simulink model "simulator"  (R2020b)
settings: Solver=FixedStepAuto  StartTime=0.0  StopTime=t_end  FixedStep=0.01  RelTol=1e-3
values from neighbouring files (symbols this model uses):
  A = zeros(6,6)    [main_simulator.m]    (also in main_simulatorTOF.m)
  B = zeros(6,3)    [main_simulator.m]    (also in main_simulatorTOF.m)
  C = zeros(3,6)    [main_simulator.m]    (also in main_simulatorTOF.m)
  D = zeros(3,3)    [main_simulator.m]    (also in main_simulatorTOF.m)
  d_input = 0*1    (= 0)    [main_simulator.m]    (also in main_simulatorTOF.m = 1)
  d_sensor = 0    [main_simulator.m]    (also in main_simulatorTOF.m)
  I = m*Rbot*Rbot/2    (= 0.3125)    [main_simulator.m]    (also in main_simulatorTOF.m)
  Kdth = 5    [main_simulator.m]    (also in main_simulatorTOF.m)
  Kdx = 80    [main_simulator.m]    (also in main_simulatorTOF.m)
  Kdy = 60    [main_simulator.m]    (also in main_simulatorTOF.m)
  Kpth = 20    [main_simulator.m]    (also in main_simulatorTOF.m)
  Kpx = 25    [main_simulator.m]    (also in main_simulatorTOF.m)
  Kpy = 10    [main_simulator.m]    (also in main_simulatorTOF.m)
  m = 10    [main_simulator.m]    (also in main_simulatorTOF.m)
  Rdist = Lw + xset    (= 0.5)    [main_simulator.m]    (also in main_simulatorTOF.m)
  X0 = zeros(6,1)    [main_simulator.m]    (also in main_simulatorTOF.m)
undefined symbols (not defined in the file or in its folder): magnitude, sigbuilder_block
libraries: simulink x3
settings Model: Creator=danny  LastModifiedBy=danny
settings SolverCC: AlgebraicLoopSolver=Auto
settings DebuggingCC: SFMachineParentedDataDiag=error

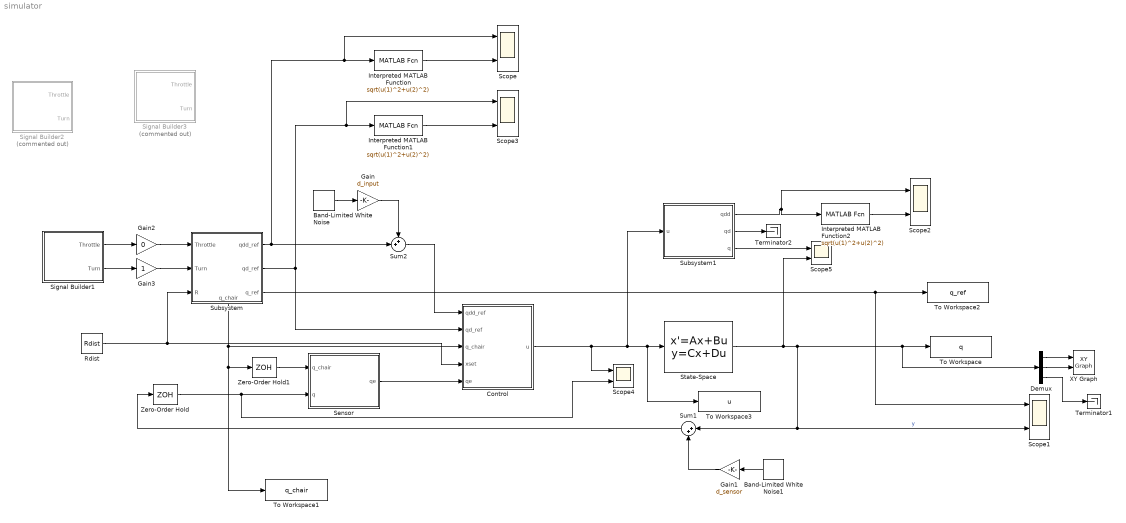
== system simulator ==
  Band-Limited White Noise : simulink/Sources/Band-Limited White Noise  Cov=[0.001]  Ts=0.1  seed=[23341]
  Band-Limited White Noise1 : simulink/Sources/Band-Limited White Noise  Cov=[0.0001]  Ts=0.15  seed=[23341]
  Control : Subsystem
  Demux : Demux  Outputs=3
  Gain : Gain  Gain=d_input
  Gain1 : Gain  Gain=d_sensor
  Gain2 : Gain  Gain=0
  Gain3 : Gain
  Interpreted MATLAB Function : MATLABFcn  MATLABFcn=sqrt(u(1)^2+u(2)^2)
  Interpreted MATLAB Function1 : MATLABFcn  MATLABFcn=sqrt(u(1)^2+u(2)^2)
  Interpreted MATLAB Function2 : MATLABFcn  MATLABFcn=sqrt(u(1)^2+u(2)^2)
  Rdist : Constant  Value=Rdist
  Scope{,1..5} (6 alike) : Scope  NumInputPorts=2
  Sensor : Subsystem
  Signal Builder1 : Subsystem  Tag=STV Subsys  LoadFcn=sigbuilder_block('load');  StartFcn=sigbuilder_block('start');  StopFcn=sigbuilder_block('stop');  ClipboardFcn=sigbuilder_block('clipboard');  mask(Sigbuilder block){tuvar=[0:10]}
      mask help: Simulink:masks:SigbuilderBlock_MD
      mask init:
      | if ~strcmp(get_param(bdroot(gcbh),'SimulationStatus'),'stopped') tuvar = sigbuilder_block('maskInit'); end
      settings: CopyFcn=sigbuilder_block('copy');  DeleteFcn=sigbuilder_block('delete');  ModelCloseFcn=sigbuilder_block('modelClose');  PreSaveFcn=sigbuilder_block('preSave');  PauseFcn=sigbuilder_block('pause');  ContinueFcn=sigbuilder_block('continue');  NameChangeFcn=sigbuilder_block('namechange');  OpenFcn=sigbuilder_block('open',[1440 169 815 516 ]);  CloseFcn=sigbuilder_block('close');
      mask Display: plot(0, 0, 100, 100,[2, 2, 32, 32, 2], [68, 8, 8, 68, 68],[32, 2], [38, 38], [32, 19, 2],[53, 60, 44], [32, 17, 17, 2],[16, 16, 31, 31]);txt = getActiveGroup(gcbh);text(2, 100, txt,'verticalAlignment', 'top');
  Signal Builder2 : Subsystem  Tag=STV Subsys  Commented=on  LoadFcn=sigbuilder_block('load');  StartFcn=sigbuilder_block('start');  StopFcn=sigbuilder_block('stop');  ClipboardFcn=sigbuilder_block('clipboard');  mask(Sigbuilder block){tuvar=[0:10]}
      mask help: Simulink:masks:SigbuilderBlock_MD
      mask init:
      | if ~strcmp(get_param(bdroot(gcbh),'SimulationStatus'),'stopped') tuvar = sigbuilder_block('maskInit'); end
      settings: CopyFcn=sigbuilder_block('copy');  DeleteFcn=sigbuilder_block('delete');  ModelCloseFcn=sigbuilder_block('modelClose');  PreSaveFcn=sigbuilder_block('preSave');  PauseFcn=sigbuilder_block('pause');  ContinueFcn=sigbuilder_block('continue');  NameChangeFcn=sigbuilder_block('namechange');  OpenFcn=sigbuilder_block('open',[87 196 1164 589 ]);  CloseFcn=sigbuilder_block('close');
      mask Display: plot(0, 0, 100, 100,[2, 2, 32, 32, 2], [68, 8, 8, 68, 68],[32, 2], [38, 38], [32, 19, 2],[53, 60, 44], [32, 17, 17, 2],[16, 16, 31, 31]);txt = getActiveGroup(gcbh);text(2, 100, txt,'verticalAlignment', 'top');
  Signal Builder3 : Subsystem  Tag=STV Subsys  Commented=on  LoadFcn=sigbuilder_block('load');  StartFcn=sigbuilder_block('start');  StopFcn=sigbuilder_block('stop');  ClipboardFcn=sigbuilder_block('clipboard');  mask(Sigbuilder block){tuvar=[0:10]}
      mask help: Simulink:masks:SigbuilderBlock_MD
      mask init:
      | if ~strcmp(get_param(bdroot(gcbh),'SimulationStatus'),'stopped') tuvar = sigbuilder_block('maskInit'); end
      settings: CopyFcn=sigbuilder_block('copy');  DeleteFcn=sigbuilder_block('delete');  ModelCloseFcn=sigbuilder_block('modelClose');  PreSaveFcn=sigbuilder_block('preSave');  PauseFcn=sigbuilder_block('pause');  ContinueFcn=sigbuilder_block('continue');  NameChangeFcn=sigbuilder_block('namechange');  OpenFcn=sigbuilder_block('open',[276 189 1164 538 ]);  CloseFcn=sigbuilder_block('close');
      mask Display: plot(0, 0, 100, 100,[2, 2, 32, 32, 2], [68, 8, 8, 68, 68],[32, 2], [38, 38], [32, 19, 2],[53, 60, 44], [32, 17, 17, 2],[16, 16, 31, 31]);txt = getActiveGroup(gcbh);text(2, 100, txt,'verticalAlignment', 'top');
  State-Space : StateSpace  A=A  B=B  C=C  D=D  InitialCondition=X0
  Subsystem : Subsystem
      settings: PortSchema="{\"entries\":[{\"content\":{\"sides\":[{\"content\":{\"connectorIds\":[\"In1\",\"In2\",\"In3\"]},\"type\":\"ConnectorPlacement.EquallySpacedRectSide\",\"uuid\":\"9e6ae883-37f6-4f77-95d7-869cca068091\"},{\"content\":{\"connectorIds\":[\"Out1\",\"Out2\",\"Out3\"],\"side\":\"RIGHT\"},\"type\":\"ConnectorPlacement.EquallySpacedRectSide\",\"uuid\":\"8baff953-0ce1-4c38-a8bf-b2873ef572e6\"},{\"content\":{\"connectorIds\":[],\"side\":\"TOP\"},\"type\":\"ConnectorPlacement.EquallySpacedRectSide\",\"uuid\":\"29b65c75-e630-4a34-89d5-db1d2bd63028\"},{\"content\":{\"connectorIds\":[\"Out4\"],\"side\":\"BOTTOM\"},\"type\":\"ConnectorPlacement.EquallySpacedRectSide\",\"uuid\":\"cc16174a-4e4f-4e75-a806-17e54c552ac2\"}]},\"type\":\"ConnectorPlacement.EquallySpacedConnector\",\"uuid\":\"f8d4b503-c69c-4ee3-88e0-362a77e21b1f\"}],\"packageUris\":[\"http://schema.mathworks.com/mf0/Connector/R2020b\"],\"version\":\"1.0\"}"
  Subsystem1 : Subsystem
  Sum1 : Sum  Inputs=|++
  Sum2 : Sum  Inputs=++|
  Terminator1 : Terminator
  Terminator2 : Terminator
  To Workspace : ToWorkspace  VariableName=q  SaveFormat=Timeseries  SampleTime=-1
  To Workspace1 : ToWorkspace  VariableName=q_chair  SaveFormat=Timeseries  SampleTime=-1
  To Workspace2 : ToWorkspace  VariableName=q_ref  SaveFormat=Timeseries  SampleTime=-1
  To Workspace3 : ToWorkspace  VariableName=u  SaveFormat=Timeseries  SampleTime=-1
  XY Graph : simulink/Sinks/XY Graph  xmin=-5  xmax=5  ymin=-5  ymax=5  st=-1
  Zero-Order Hold : ZeroOrderHold  SampleTime=0.15
  Zero-Order Hold1 : ZeroOrderHold  SampleTime=0.15
  wires:
  State-Space/1 -> Scope5/2, Demux/1, To Workspace/1, Scope1/2, Sum1/1  "y"
  Rdist/1 -> Subsystem/3(R), Control/4(xset)
  Band-Limited White Noise/1 -> Gain/1
  Gain/1 -> Sum2/1
  Band-Limited White Noise1/1 -> Gain1/1
  Gain1/1 -> Sum1/2
  Subsystem/3(q_ref) -> Scope1/1, To Workspace2/1
  Subsystem/1(qdd_ref) -> Scope/1, Interpreted MATLAB Function/1, Sum2/2
  Subsystem/4(q_chair) -> Zero-Order Hold1/1, To Workspace1/1, Control/3(q_chair)
  Subsystem/2(qd_ref) -> Control/2(qd_ref), Scope3/1, Interpreted MATLAB Function1/1
  Signal Builder1/1(Throttle) -> Gain2/1
  Sum1/1 -> Zero-Order Hold/1
  Interpreted MATLAB Function/1 -> Scope/2
  Interpreted MATLAB Function1/1 -> Scope3/2
  Sum2/1 -> Control/1(qdd_ref)
  Sensor/1(qe) -> Control/5(qe)
  Control/1(u) -> Scope4/1, State-Space/1, To Workspace3/1, Subsystem1/1(u)
  Subsystem1/3(q) -> Scope5/1
  Zero-Order Hold/1 -> Scope4/2, Sensor/2(q)
  Zero-Order Hold1/1 -> Sensor/1(q_chair)
  Demux/1 -> XY Graph/1
  Demux/3 -> Terminator1/1
  Demux/2 -> XY Graph/2
  Interpreted MATLAB Function2/1 -> Scope2/2
  Subsystem1/1(qdd) -> Scope2/1, Interpreted MATLAB Function2/1
  Subsystem1/2(qd) -> Terminator2/1
  Gain2/1 -> Subsystem/1(Throttle)
  Gain3/1 -> Subsystem/2(Turn)
  Signal Builder1/2(Turn) -> Gain3/1

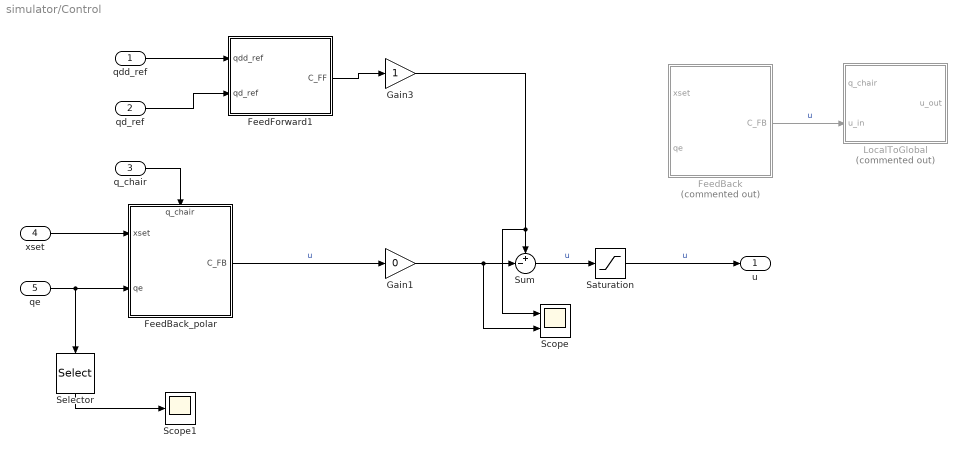
== system simulator/Control ==
  qdd_ref : Inport
  qd_ref : Inport  Port=2
  q_chair : Inport  Port=3
  xset : Inport  Port=4
  qe : Inport  Port=5
  FeedBack : Subsystem  Commented=on
  FeedBack_polar : Subsystem
      settings: PortSchema="{\"entries\":[{\"content\":{\"sides\":[{\"content\":{\"connectorIds\":[\"In1\",\"In2\"]},\"type\":\"ConnectorPlacement.EquallySpacedRectSide\",\"uuid\":\"cbe067bd-6f36-47e3-b114-7ad219aeaebc\"},{\"content\":{\"connectorIds\":[\"Out1\"],\"side\":\"RIGHT\"},\"type\":\"ConnectorPlacement.EquallySpacedRectSide\",\"uuid\":\"c93f1609-f1ce-4d77-9628-c6a9c4217eec\"},{\"content\":{\"connectorIds\":[\"In3\"],\"side\":\"TOP\"},\"type\":\"ConnectorPlacement.EquallySpacedRectSide\",\"uuid\":\"a9439a30-db70-4f29-82a3-671799b82d8c\"}]},\"type\":\"ConnectorPlacement.EquallySpacedConnector\",\"uuid\":\"d7bf9452-d630-4580-9a6c-30f601efa431\"}],\"packageUris\":[\"http://schema.mathworks.com/mf0/Connector/R2020b\"],\"version\":\"1.0\"}"
  FeedForward1 : Subsystem
  Gain1 : Gain  Gain=0
  Gain3 : Gain
  LocalToGlobal : Subsystem  Commented=on
  Saturation : Saturate  UpperLimit=15  LowerLimit=-15
  Scope : Scope  NumInputPorts=2
  Scope1 : Scope
  Selector : Selector  InputPortWidth=3  IndexOptions=Index vector (dialog)  Indices=[1 2]  OutputSizes=1
  Sum : Sum  Inputs=+-|
  u : Outport
  wires:
  Sum/1 -> Saturation/1  "u"
  xset/1 -> FeedBack_polar/1(xset)
  Gain3/1 -> Scope/1, Sum/1
  qdd_ref/1 -> FeedForward1/1(qdd_ref)
  FeedForward1/1(C_FF) -> Gain3/1
  Gain1/1 -> Scope/2, Sum/2
  Saturation/1 -> u/1  "u"
  FeedBack/1(C_FB) -> LocalToGlobal/2(u_in)  "u"
  qe/1 -> FeedBack_polar/2(qe), Selector/1
  q_chair/1 -> FeedBack_polar/3(q_chair)
  FeedBack_polar/1(C_FB) -> Gain1/1  "u"
  Selector/1 -> Scope1/1
  qd_ref/1 -> FeedForward1/2(qd_ref)

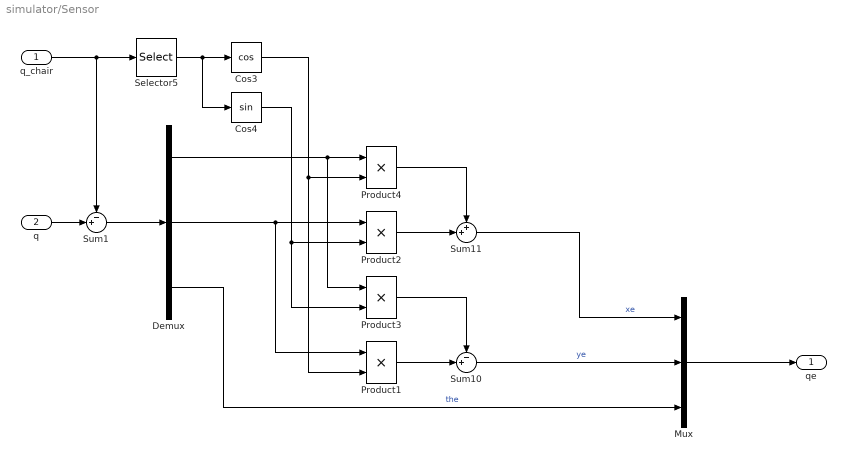
== system simulator/Sensor ==
  q_chair : Inport
  q : Inport  Port=2
  Cos3 : Trigonometry  Operator=cos
  Cos4 : Trigonometry
  Demux : Demux  Outputs=3
  Mux : Mux  Inputs=3
  Product{1..4} (4 alike) : Product
  Selector5 : Selector  InputPortWidth=3  IndexOptions=Index vector (dialog)  Indices=[3]  OutputSizes=1
  Sum1 : Sum  Inputs=-+|
  Sum10 : Sum  Inputs=-+|
  Sum11 : Sum  Inputs=++|
  qe : Outport
  wires:
  Selector5/1 -> Cos4/1, Cos3/1
  Sum11/1 -> Mux/1  "xe"
  Sum10/1 -> Mux/2  "ye"
  Product1/1 -> Sum10/2
  Product3/1 -> Sum10/1
  Demux/2 -> Product2/1, Product1/1
  Demux/1 -> Product3/1, Product4/1
  Product4/1 -> Sum11/1
  Product2/1 -> Sum11/2
  Cos3/1 -> Product4/2, Product1/2
  Cos4/1 -> Product2/2, Product3/2
  Sum1/1 -> Demux/1
  q_chair/1 -> Sum1/1, Selector5/1
  q/1 -> Sum1/2
  Demux/3 -> Mux/3  "the"
  Mux/1 -> qe/1

== system simulator/Signal Builder1 ==
  Demux : Demux  Tag=STV Demux  Outputs=2
      settings: DisplayOption=none
  FromWs : FromWorkspace  Tag=STV FromWs  VariableName=tuvar
      SigBuilderData=|
      | common.afterFinalStr = 'Extrapolate'
      | common.sampleTime = 0
      | dataSet.timeRange = [0 20]
      | dataSet.name = 'Group 1'
      | sbobj.Groups.Name = 'Group 1'
      | sbobj.Groups.Signals(1).Name = 'Throttle'
      | sbobj.Groups.Signals(1).XData = [0 3 3 6 6 7 7 10 10 17.1 17.1 18.1 18.1 19.1 19.1 20]
      | sbobj.Groups.Signals(1).YData = [0 0 1.5 1.5 0 0 -1.5 -1.5 0 0 1 1 -1 -1 0 0]
      | sbobj.Groups.Signals(2).Name = 'Turn'
      | sbobj.Groups.Signals(2).XData = [0 0.5 0.5 1.25 1.25 2 2 10 10 11 11 15 15 16 16 20]
      | sbobj.Groups.Signals(2).YData = [0 0 3.5 3.5 -3.5 -3.5 0 0 1 1 0 0 -1 -1 0 0]
      | sbobj.Groups.TimeRange = [0 20]
  Throttle : Outport  Tag=STV Outport
  Turn : Outport  Tag=STV Outport  Port=2
  wires:
  Demux/1 -> Throttle/1
  FromWs/1 -> Demux/1
  Demux/2 -> Turn/1

== system simulator/Signal Builder2 ==
  Demux : Demux  Tag=STV Demux  Outputs=2
      settings: DisplayOption=none
  FromWs : FromWorkspace  Tag=STV FromWs  VariableName=tuvar
      SigBuilderData=|
      | common.afterFinalStr = 'Extrapolate'
      | common.sampleTime = 0
      | dataSet.timeRange = [0 20]
      | dataSet.name = 'Group 1'
      | sbobj.Groups.Name = 'Group 1'
      | sbobj.Groups.Signals(1).Name = 'Throttle'
      | sbobj.Groups.Signals(1).XData = [0 3.1 20]
      | sbobj.Groups.Signals(1).YData = [0 0 0]
      | sbobj.Groups.Signals(2).Name = 'Turn'
      | sbobj.Groups.Signals(2).XData = [0 0.5 1 1.5 7 7.5 8 20]
      | sbobj.Groups.Signals(2).YData = [0 0 0.9 0 0 -0.9 0 0]
      | sbobj.Groups.TimeRange = [0 20]
  Throttle : Outport  Tag=STV Outport
  Turn : Outport  Tag=STV Outport  Port=2
  wires:
  Demux/2 -> Turn/1
  FromWs/1 -> Demux/1
  Demux/1 -> Throttle/1

== system simulator/Signal Builder3 ==
  Demux : Demux  Tag=STV Demux  Outputs=2
      settings: DisplayOption=none
  FromWs : FromWorkspace  Tag=STV FromWs  VariableName=tuvar
      SigBuilderData=|
      | common.afterFinalStr = 'Extrapolate'
      | common.sampleTime = 0
      | dataSet.timeRange = [0 20]
      | dataSet.name = 'Group 1'
      | sbobj.Groups.Name = 'Group 1'
      | sbobj.Groups.Signals(1).Name = 'Throttle'
      | sbobj.Groups.Signals(1).XData = [0 3.1 20]
      | sbobj.Groups.Signals(1).YData = [0 0 0]
      | sbobj.Groups.Signals(2).Name = 'Turn'
      | sbobj.Groups.Signals(2).XData = [0 0.5 1 1.5 7 7.5 8 12 12 12.75 12.75 13.5 13.5 20]
      | sbobj.Groups.Signals(2).YData = [0 0 0.2 0 0 -0.2 0 0 -3.5 -3.5 3.5 3.5 0 0]
      | sbobj.Groups.TimeRange = [0 20]
  Throttle : Outport  Tag=STV Outport
  Turn : Outport  Tag=STV Outport  Port=2
  wires:
  Demux/1 -> Throttle/1
  FromWs/1 -> Demux/1
  Demux/2 -> Turn/1

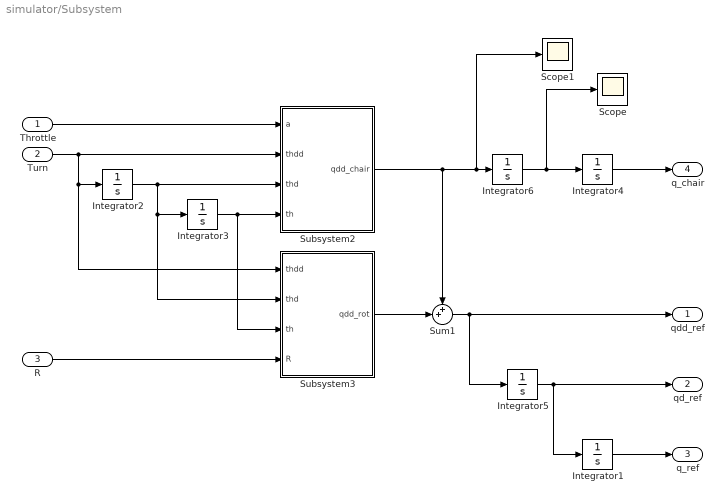
== system simulator/Subsystem ==
  Throttle : Inport
  Turn : Inport  Port=2
  R : Inport  Port=3
  Integrator1 : Integrator  InitialCondition=X0ref(2:2:end)
  Integrator{2..6} (5 alike) : Integrator
  Scope : Scope
  Scope1 : Scope
  Subsystem2 : Subsystem
  Subsystem3 : Subsystem
  Sum1 : Sum  Inputs=++|
  qdd_ref : Outport
  qd_ref : Outport  Port=2
  q_ref : Outport  Port=3
  q_chair : Outport  Port=4
  wires:
  Integrator2/1 -> Subsystem3/2(thd), Integrator3/1, Subsystem2/3(thd)
  Integrator1/1 -> q_ref/1
  Sum1/1 -> qdd_ref/1, Integrator5/1
  Integrator4/1 -> q_chair/1
  Subsystem2/1(qdd_chair) -> Sum1/1, Scope1/1, Integrator6/1
  Throttle/1 -> Subsystem2/1(a)
  Integrator3/1 -> Subsystem3/3(th), Subsystem2/4(th)
  Turn/1 -> Subsystem3/1(thdd), Integrator2/1, Subsystem2/2(thdd)
  Subsystem3/1(qdd_rot) -> Sum1/2
  Integrator5/1 -> qd_ref/1, Integrator1/1
  R/1 -> Subsystem3/4(R)
  Integrator6/1 -> Scope/1, Integrator4/1

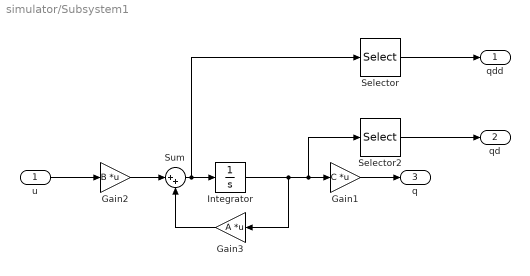
== system simulator/Subsystem1 ==
  u : Inport
  Gain1 : Gain  Gain=C  Multiplication=Matrix(K*u)
  Gain2 : Gain  Gain=B  Multiplication=Matrix(K*u)
  Gain3 : Gain  Gain=A  Multiplication=Matrix(K*u)
  Integrator : Integrator  InitialCondition=X0
  Selector : Selector  InputPortWidth=6  IndexOptions=Index vector (dialog)  Indices=[1 3]  OutputSizes=1
  Selector2 : Selector  InputPortWidth=6  IndexOptions=Index vector (dialog)  Indices=[1 3 5]  OutputSizes=1
  Sum : Sum  Inputs=|++
  qdd : Outport
  qd : Outport  Port=2
  q : Outport  Port=3
  wires:
  Gain1/1 -> q/1
  u/1 -> Gain2/1
  Integrator/1 -> Gain3/1, Selector2/1, Gain1/1
  Sum/1 -> Selector/1, Integrator/1
  Gain2/1 -> Sum/1
  Gain3/1 -> Sum/2
  Selector2/1 -> qd/1
  Selector/1 -> qdd/1

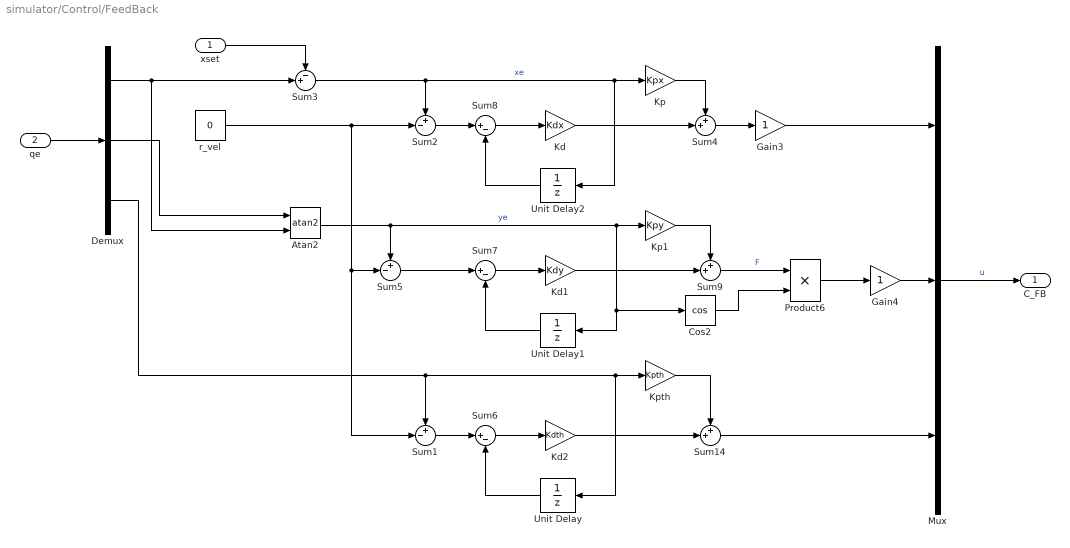
== system simulator/Control/FeedBack ==
  xset : Inport
  qe : Inport  Port=2
  Atan2 : Trigonometry  Operator=atan2
  Cos2 : Trigonometry  Operator=cos
  Demux : Demux  Outputs=3
  Gain3 : Gain
  Gain4 : Gain
  Kd : Gain  Gain=Kdx
  Kd1 : Gain  Gain=Kdy
  Kd2 : Gain  Gain=Kdth
  Kp : Gain  Gain=Kpx
  Kp1 : Gain  Gain=Kpy
  Kpth : Gain  Gain=Kpth
  Mux : Mux  Inputs=3
  Product6 : Product
  Sum1 : Sum  Inputs=+-|
  Sum14 : Sum  Inputs=++|
  Sum2 : Sum  Inputs=+-|
  Sum3 : Sum  Inputs=-+|
  Sum4 : Sum  Inputs=++|
  Sum5 : Sum  Inputs=+-|
  Sum6 : Sum  Inputs=|+-
  Sum7 : Sum  Inputs=|+-
  Sum8 : Sum  Inputs=|+-
  Sum9 : Sum  Inputs=++|
  Unit Delay : UnitDelay  SampleTime=-1  HasFrameUpgradeWarning=on
  Unit Delay1 : UnitDelay  SampleTime=-1  HasFrameUpgradeWarning=on
  Unit Delay2 : UnitDelay  SampleTime=-1  HasFrameUpgradeWarning=on
  r_vel : Constant  Value=0
  C_FB : Outport
  wires:
  Kd/1 -> Sum4/2
  Mux/1 -> C_FB/1  "u"
  Kp1/1 -> Sum9/1
  Kd1/1 -> Sum9/2
  xset/1 -> Sum3/1
  Sum3/1 -> Unit Delay2/1, Kp/1, Sum2/1  "xe"
  Kp/1 -> Sum4/1
  Kpth/1 -> Sum14/1
  Sum14/1 -> Mux/3
  Demux/3 -> Sum1/1, Unit Delay/1, Kpth/1
  Unit Delay/1 -> Sum6/2
  r_vel/1 -> Sum2/2, Sum5/2, Sum1/2
  Sum6/1 -> Kd2/1
  Sum1/1 -> Sum6/1
  Kd2/1 -> Sum14/2
  Sum5/1 -> Sum7/1
  Unit Delay1/1 -> Sum7/2
  Sum8/1 -> Kd/1
  Unit Delay2/1 -> Sum8/2
  Sum2/1 -> Sum8/1
  Product6/1 -> Gain4/1
  Sum4/1 -> Gain3/1
  qe/1 -> Demux/1
  Cos2/1 -> Product6/2
  Sum9/1 -> Product6/1  "F"
  Gain3/1 -> Mux/1
  Gain4/1 -> Mux/2
  Sum7/1 -> Kd1/1
  Demux/2 -> Atan2/1
  Atan2/1 -> Unit Delay1/1, Cos2/1, Kp1/1, Sum5/1  "ye"
  Demux/1 -> Sum3/2, Atan2/2

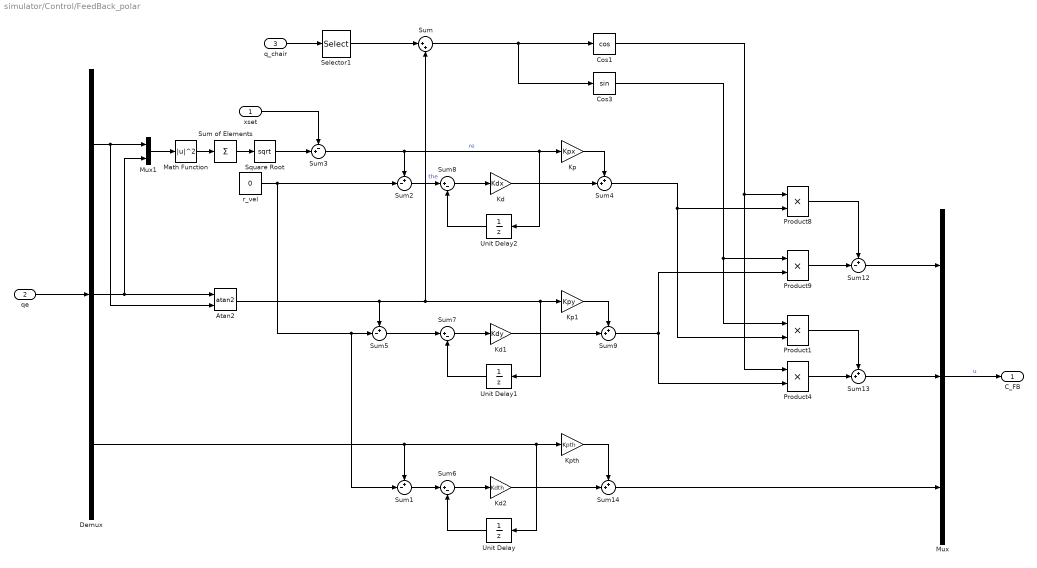
== system simulator/Control/FeedBack_polar ==
  xset : Inport
  qe : Inport  Port=2
  q_chair : Inport  Port=3
  Atan2 : Trigonometry  Operator=atan2
  Cos1 : Trigonometry  Operator=cos
  Cos3 : Trigonometry
  Demux : Demux  Outputs=3
  Kd : Gain  Gain=Kdx
  Kd1 : Gain  Gain=Kdy
  Kd2 : Gain  Gain=Kdth
  Kp : Gain  Gain=Kpx
  Kp1 : Gain  Gain=Kpy
  Kpth : Gain  Gain=Kpth
  Math Function : Math  Operator=magnitude^2  SaturateOnIntegerOverflow=on
  Mux : Mux  Inputs=3
  Mux1 : Mux  Inputs=2
  Product{1,4,8..9} (4 alike) : Product
  Selector1 : Selector  InputPortWidth=3  IndexOptions=Index vector (dialog)  Indices=[3]  OutputSizes=1
  Square Root : Sqrt  SaturateOnIntegerOverflow=on
  Sum : Sum  Inputs=|++
  Sum of Elements : Sum  Inputs=+
  Sum{1..2,5,12} (4 alike) : Sum  Inputs=+-|
  Sum{4,9,13..14} (4 alike) : Sum  Inputs=++|
  Sum3 : Sum  Inputs=-+|
  Sum6 : Sum  Inputs=|+-
  Sum7 : Sum  Inputs=|+-
  Sum8 : Sum  Inputs=|+-
  Unit Delay : UnitDelay  SampleTime=-1  HasFrameUpgradeWarning=on
  Unit Delay1 : UnitDelay  SampleTime=-1  HasFrameUpgradeWarning=on
  Unit Delay2 : UnitDelay  SampleTime=-1  HasFrameUpgradeWarning=on
  r_vel : Constant  Value=0
  C_FB : Outport
  wires:
  Kd/1 -> Sum4/2
  Mux/1 -> C_FB/1  "u"
  Kp1/1 -> Sum9/1
  Kd1/1 -> Sum9/2
  Sum3/1 -> Unit Delay2/1, Kp/1, Sum2/1  "re"
  Kp/1 -> Sum4/1
  Kpth/1 -> Sum14/1
  Sum14/1 -> Mux/3
  Demux/3 -> Unit Delay/1, Kpth/1, Sum1/1
  Unit Delay/1 -> Sum6/2
  r_vel/1 -> Sum2/2, Sum5/2, Sum1/2
  Sum6/1 -> Kd2/1
  Sum1/1 -> Sum6/1
  Kd2/1 -> Sum14/2
  Sum5/1 -> Sum7/1
  Unit Delay1/1 -> Sum7/2
  Sum8/1 -> Kd/1
  Unit Delay2/1 -> Sum8/2
  Sum2/1 -> Sum8/1
  qe/1 -> Demux/1
  Sum9/1 -> Product9/2, Product4/2
  Product9/1 -> Sum12/2
  Sum7/1 -> Kd1/1
  Demux/2 -> Mux1/2, Atan2/1
  Atan2/1 -> Sum5/1, Sum/2, Unit Delay1/1, Kp1/1  "the"
  Demux/1 -> Mux1/1, Atan2/2
  q_chair/1 -> Selector1/1
  Math Function/1 -> Sum of Elements/1
  Sum of Elements/1 -> Square Root/1
  Mux1/1 -> Math Function/1
  Square Root/1 -> Sum3/2
  Sum4/1 -> Product1/2, Product8/2
  Cos3/1 -> Product9/1, Product1/1
  Cos1/1 -> Product4/1, Product8/1
  Product4/1 -> Sum13/2
  Sum/1 -> Cos3/1, Cos1/1
  Sum13/1 -> Mux/2
  xset/1 -> Sum3/1
  Sum12/1 -> Mux/1
  Selector1/1 -> Sum/1
  Product8/1 -> Sum12/1
  Product1/1 -> Sum13/1

== system simulator/Control/FeedForward1 ==
  qdd_ref : Inport
  qd_ref : Inport  Port=2
  Gain1 : Gain  Gain=m
  Gain2 : Gain  Commented=on  Gain=I
  Mux : Mux  Inputs=2
  Selector : Selector  InputPortWidth=3  IndexOptions=Index vector (dialog)  Indices=[1 2]  OutputSizes=1
  Selector1 : Selector  InputPortWidth=3  IndexOptions=Index vector (dialog)  Indices=[3]  OutputSizes=1
  C_FF : Outport
  wires:
  Mux/1 -> C_FF/1
  Gain1/1 -> Mux/1  "u"
  Selector/1 -> Gain1/1
  qdd_ref/1 -> Selector/1
  qd_ref/1 -> Selector1/1
  Selector1/1 -> Mux/2

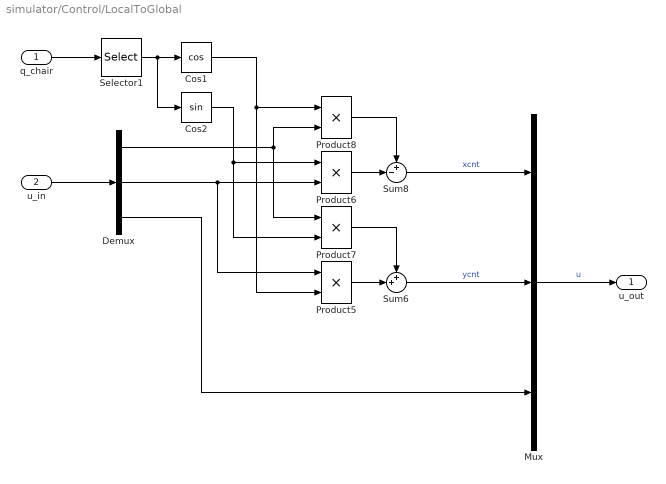
== system simulator/Control/LocalToGlobal ==
  q_chair : Inport
  u_in : Inport  Port=2
  Cos1 : Trigonometry  Operator=cos
  Cos2 : Trigonometry
  Demux : Demux  Outputs=3
  Mux : Mux  Inputs=3
  Product{5..8} (4 alike) : Product
  Selector1 : Selector  InputPortWidth=3  IndexOptions=Index vector (dialog)  Indices=[3]  OutputSizes=1
  Sum6 : Sum  Inputs=++|
  Sum8 : Sum  Inputs=+-|
  u_out : Outport
  wires:
  Demux/2 -> Product6/2, Product5/1
  Sum6/1 -> Mux/2  "ycnt"
  Product6/1 -> Sum8/2
  Sum8/1 -> Mux/1  "xcnt"
  Demux/1 -> Product8/2, Product7/1
  q_chair/1 -> Selector1/1
  Cos1/1 -> Product5/2, Product8/1
  Product5/1 -> Sum6/2
  Cos2/1 -> Product7/2, Product6/1
  Product7/1 -> Sum6/1
  Selector1/1 -> Cos2/1, Cos1/1
  Product8/1 -> Sum8/1
  Mux/1 -> u_out/1  "u"
  u_in/1 -> Demux/1
  Demux/3 -> Mux/3

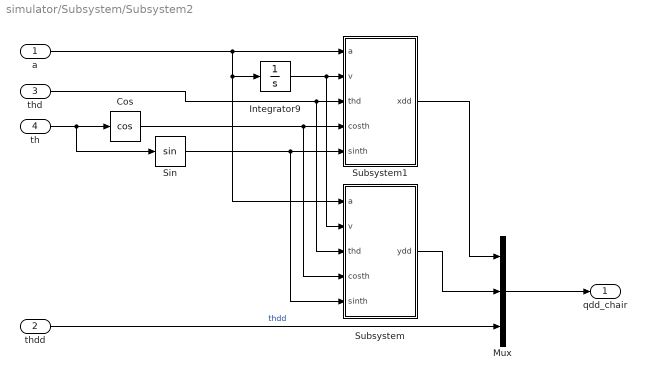
== system simulator/Subsystem/Subsystem2 ==
  a : Inport
  thdd : Inport  Port=2
  thd : Inport  Port=3
  th : Inport  Port=4
  Cos : Trigonometry  Operator=cos
  Integrator9 : Integrator
  Mux : Mux  Inputs=3
  Sin : Trigonometry
  Subsystem : Subsystem
  Subsystem1 : Subsystem
  qdd_chair : Outport
  wires:
  Cos/1 -> Subsystem/4(costh), Subsystem1/4(costh)
  th/1 -> Cos/1, Sin/1
  Mux/1 -> qdd_chair/1
  thdd/1 -> Mux/3  "thdd"
  thd/1 -> Subsystem/3(thd), Subsystem1/3(thd)
  Sin/1 -> Subsystem1/5(sinth), Subsystem/5(sinth)
  a/1 -> Subsystem1/1(a), Subsystem/1(a), Integrator9/1
  Integrator9/1 -> Subsystem1/2(v), Subsystem/2(v)
  Subsystem/1(ydd) -> Mux/2
  Subsystem1/1(xdd) -> Mux/1

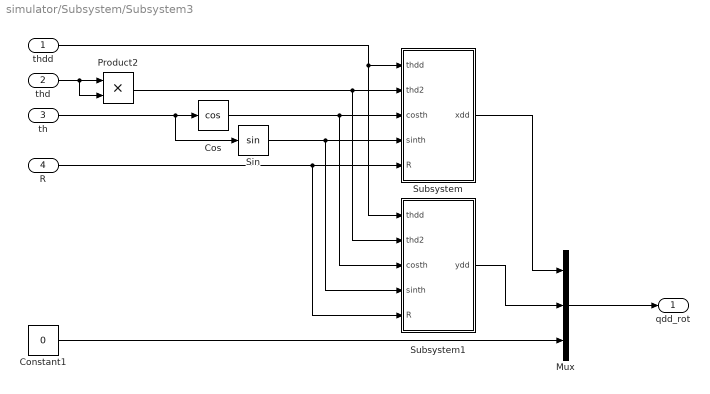
== system simulator/Subsystem/Subsystem3 ==
  thdd : Inport
  thd : Inport  Port=2
  th : Inport  Port=3
  R : Inport  Port=4
  Constant1 : Constant  Value=0
  Cos : Trigonometry  Operator=cos
  Mux : Mux  Inputs=3
  Product2 : Product
  Sin : Trigonometry
  Subsystem : Subsystem
  Subsystem1 : Subsystem
  qdd_rot : Outport
  wires:
  thdd/1 -> Subsystem1/1(thdd), Subsystem/1(thdd)
  thd/1 -> Product2/1, Product2/2
  th/1 -> Sin/1, Cos/1
  Sin/1 -> Subsystem/4(sinth), Subsystem1/4(sinth)
  Cos/1 -> Subsystem/3(costh), Subsystem1/3(costh)
  Mux/1 -> qdd_rot/1
  Product2/1 -> Subsystem1/2(thd2), Subsystem/2(thd2)
  R/1 -> Subsystem1/5(R), Subsystem/5(R)
  Subsystem/1(xdd) -> Mux/1
  Subsystem1/1(ydd) -> Mux/2
  Constant1/1 -> Mux/3

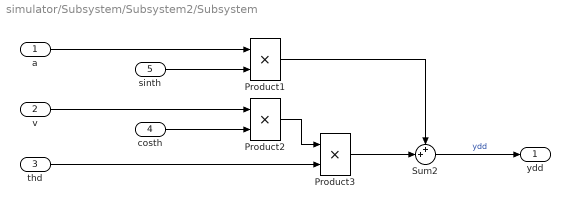
== system simulator/Subsystem/Subsystem2/Subsystem ==
  a : Inport
  v : Inport  Port=2
  thd : Inport  Port=3
  costh : Inport  Port=4
  sinth : Inport  Port=5
  Product1 : Product
  Product2 : Product
  Product3 : Product
  Sum2 : Sum  Inputs=++|
  ydd : Outport
  wires:
  costh/1 -> Product2/2
  Sum2/1 -> ydd/1  "ydd"
  Product3/1 -> Sum2/2
  Product2/1 -> Product3/1
  Product1/1 -> Sum2/1
  thd/1 -> Product3/2
  sinth/1 -> Product1/2
  a/1 -> Product1/1
  v/1 -> Product2/1

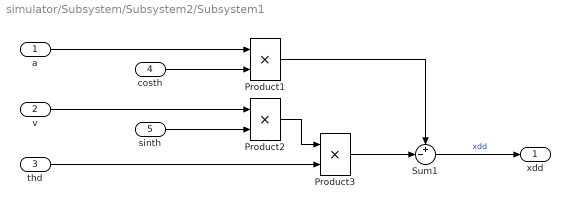
== system simulator/Subsystem/Subsystem2/Subsystem1 ==
  a : Inport
  v : Inport  Port=2
  thd : Inport  Port=3
  costh : Inport  Port=4
  sinth : Inport  Port=5
  Product1 : Product
  Product2 : Product
  Product3 : Product
  Sum1 : Sum  Inputs=+-|
  xdd : Outport
  wires:
  costh/1 -> Product1/2
  v/1 -> Product2/1
  Product1/1 -> Sum1/1
  sinth/1 -> Product2/2
  thd/1 -> Product3/2
  a/1 -> Product1/1
  Product2/1 -> Product3/1
  Sum1/1 -> xdd/1  "xdd"
  Product3/1 -> Sum1/2

== system simulator/Subsystem/Subsystem3/Subsystem ==
  thdd : Inport
  thd2 : Inport  Port=2
  costh : Inport  Port=3
  sinth : Inport  Port=4
  R : Inport  Port=5
  Product3 : Product
  Product4 : Product
  Product6 : Product
  Sum1 : Sum  Inputs=--|
  xdd : Outport
  wires:
  costh/1 -> Product4/2
  Product6/1 -> xdd/1  "xdd"
  Product4/1 -> Sum1/2
  Product3/1 -> Sum1/1
  R/1 -> Product6/2
  sinth/1 -> Product3/2
  thdd/1 -> Product3/1
  thd2/1 -> Product4/1
  Sum1/1 -> Product6/1

== system simulator/Subsystem/Subsystem3/Subsystem1 ==
  thdd : Inport
  thd2 : Inport  Port=2
  costh : Inport  Port=3
  sinth : Inport  Port=4
  R : Inport  Port=5
  Product3 : Product
  Product4 : Product
  Product6 : Product
  Sum1 : Sum  Inputs=+-|
  ydd : Outport
  wires:
  Sum1/1 -> Product6/1
  thd2/1 -> Product4/1
  thdd/1 -> Product3/1
  costh/1 -> Product3/2
  R/1 -> Product6/2
  Product3/1 -> Sum1/1
  Product4/1 -> Sum1/2
  Product6/1 -> ydd/1  "ydd"
  sinth/1 -> Product4/2
